simulink model "stimulus"  (Simulink 7.2)
settings: Solver=ode45  StartTime=0.0  StopTime=10.0  RelTol=1e-3
undefined symbols (not defined in the file or in its folder): ecgGen, emgGen, gray, scGen
libraries: dspbuff3 x3, dspsrcs4 x3, vipsrcs x1, vipsnks x1
settings Model: Creator=rafa  LastModifiedBy=rafa

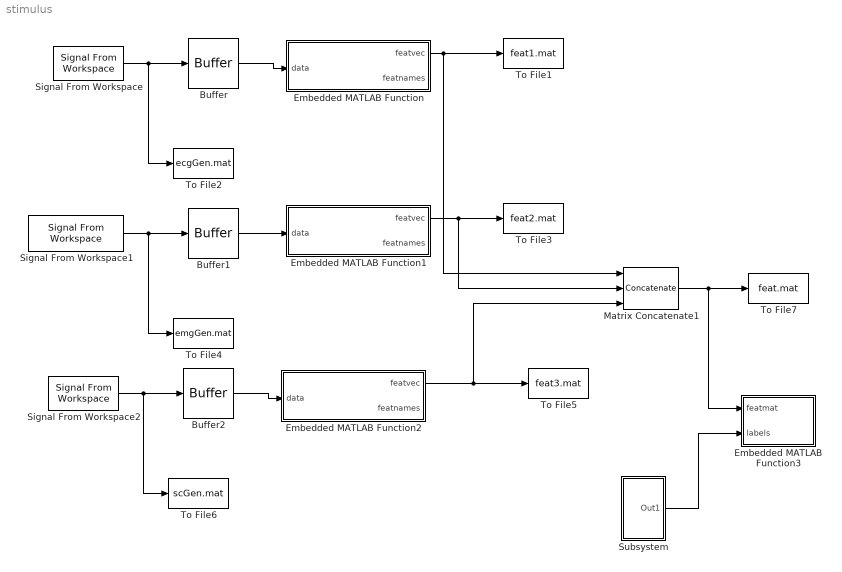
== system stimulus ==
  Buffer : dspbuff3/Buffer  N=100  V=0  ic=0
  Buffer1 : dspbuff3/Buffer  N=100  V=0  ic=0
  Buffer2 : dspbuff3/Buffer  N=100  V=0  ic=0
  Embedded MATLAB Function : Stateflow chart
  Embedded MATLAB Function1 : Stateflow chart
  Embedded MATLAB Function2 : Stateflow chart
  Embedded MATLAB Function3 : Stateflow chart
  Matrix Concatenate1 : Concatenate  NumInputs=3  Mode=Multidimensional array
  Signal From Workspace : dspsrcs4/Signal From Workspace  SystemSampleTime=-1  X=ecgGen(10)  Ts=0.001  nsamps=1  OutputAfterFinalValue=Setting to zero  ignoreOrWarnInputAndFrameLengths=off
  Signal From Workspace1 : dspsrcs4/Signal From Workspace  SystemSampleTime=-1  X=emgGen(10)  Ts=0.001  nsamps=1  OutputAfterFinalValue=Setting to zero  ignoreOrWarnInputAndFrameLengths=off
  Signal From Workspace2 : dspsrcs4/Signal From Workspace  SystemSampleTime=-1  X=scGen(10)  Ts=0.001  nsamps=1  OutputAfterFinalValue=Setting to zero  ignoreOrWarnInputAndFrameLengths=off
  Subsystem : Subsystem
  To File1 : ToFile  Filename=feat1.mat  MatrixName=ecgfeat
  To File2 : ToFile  Filename=ecgGen.mat  MatrixName=ecg
  To File3 : ToFile  Filename=feat2.mat  MatrixName=emgfeat
  To File4 : ToFile  Filename=emgGen.mat  MatrixName=emg
  To File5 : ToFile  Filename=feat3.mat  MatrixName=scfeat
  To File6 : ToFile  Filename=scGen.mat  MatrixName=sc
  To File7 : ToFile  Filename=feat.mat  MatrixName=feat
  wires:
  Signal From Workspace/1 -> Buffer/1, To File2/1
  Buffer/1 -> Embedded MATLAB Function/1(data)
  Embedded MATLAB Function/1(featvec) -> To File1/1, Matrix Concatenate1/1
  Signal From Workspace1/1 -> Buffer1/1, To File4/1
  Buffer1/1 -> Embedded MATLAB Function1/1(data)
  Embedded MATLAB Function1/1(featvec) -> To File3/1, Matrix Concatenate1/2
  Signal From Workspace2/1 -> Buffer2/1, To File6/1
  Buffer2/1 -> Embedded MATLAB Function2/1(data)
  Embedded MATLAB Function2/1(featvec) -> To File5/1, Matrix Concatenate1/3
  Matrix Concatenate1/1 -> To File7/1, Embedded MATLAB Function3/1(featmat)
  Subsystem/1(Out1) -> Embedded MATLAB Function3/2(labels)

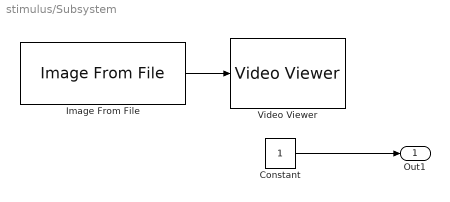
== system stimulus/Subsystem ==
  Constant : Constant  OutDataType=sfix(16)  OutScaling=2^0
  Image From File : vipsrcs/Image From File  Tag=vipblks_nd  DialogController=vipDDGCreate  DialogControllerArgs=DataTag0  SystemSampleTime=-1  FileName=/Users/rafa/MATLAB/siento/simulation/stimulus1.jpg  imagePorts=One multidimensional signal  Ts=inf  ImageDataType=Inherit from input image  Signed=on  WordLength=16  sdImageDataType=uint(8)  FractionLengthMode=User-defined  FractionLength=15  OutPortLabels=R|G|B
  Video Viewer : vipsnks/Video Viewer  DialogController=vipDDGCreate  DialogControllerArgs=DataTag1  inputType=Obsolete7b  imagePorts=One multidimensional signal  useColorMap=off  colormapValue=gray(256)  specRange=off  minInputVal=0  maxInputVal=255  FigPos=[720 739 480 640]  AxisZoom=on  trueSizedOnce=on
  Out1 : Outport  OutDataType=sfix(16)  OutScaling=2^0
  wires:
  Image From File/1 -> Video Viewer/1
  Constant/1 -> Out1/1

== matlab function Embedded MATLAB Function1 ==
  data: data input double; featvec output double; featnames output double
function [featvec,featnames] = aubt_proxy_emg(data)
% This block supports the Embedded MATLAB subset.
% See the help menu for details. 
hz=1000;
%[featvec, featnames]=aubt_extractFeatSC(data,hz);

%testing setup
featvec=[sum(data);rand(3,1)];
%simulink doesn't support string or char outputs, so convert to int
featnames=uint8(['feat1'; 'feat2'; 'feat3'; 'feat4']);

== matlab function Embedded MATLAB Function ==
  data: data input double; featvec output double; featnames output double
function [featvec,featnames]  = aubt_proxy_ecg_2(data)
% This block supports the Embedded MATLAB subset.
% See the help menu for details. 
hz=1000;
%[featvec, featnames]=aubt_extractFeatECG(data,hz);

%testing setup
featvec=[sum(data);rand(3,1)];
%simulink doesn't support string or char outputs, so convert to int
featnames=uint8(['feat1'; 'feat2'; 'feat3'; 'feat4']);

== matlab function Embedded MATLAB Function2 ==
  data: data input double; featvec output double; featnames output double
function [featvec, featnames] = aubt_proxy_ecg_2(data)
% This block supports the Embedded MATLAB subset.
% See the help menu for details. 
hz=1000;
%[featvec, featnames]=aubt_extractFeatECG(data,hz);

%testing setup
featvec=[sum(data);rand(3,1)];
%simulink doesn't support string or char outputs, so convert to int
featnames=uint8(['feat1'; 'feat2'; 'feat3'; 'feat4']);

== matlab function Embedded MATLAB Function3 ==
  data: featmat input double; labels input double
function  fisherPlot(featmat, labels)
% This block supports the Embedded MATLAB subset.
% See the help menu for details. 

eml.extrinsic('aubt_fisherPlot');
%aubt_fisherPlot(featmat,labels,'r',3,[]);
